simulink model "power_wind_dfig"  (R2016a)
settings: Solver=ode23tb  StartTime=0.0  StopTime=100  FixedStep=1/60  MaxStep=1/60  RelTol=1e-4  AbsTol=1e-3
InitFcn:
  | xInitial = init_power_wind_dfig;
undefined symbols (not defined in the file): b0, D1, D11, Delta, F, find_system, Fnom, gcbh, H, ILd_init, ILq_init, Imax_grid_conv, Init, j, Kd, Ki_dc_reg, Ki_grid_side_cur_reg, Ki_power_reg, Ki_Q, Ki_rotor_side_cur_reg, Ki_volt_reg, Kp, Kp_dc_reg, Kp_grid_side_cur_reg, Kp_power_reg, Kp_Q, Kp_rotor_side_cur_reg, Kp_volt_reg, L_RL, Llr, Lls, p, Pnom, power_A, power_B, power_D, R_RL, Rr, Rs, speed_A, speed_B, speed_C, speed_D, sps_rtmsupport, Vcontrol, Vnom, Wind_On, wo
libraries: powerlib_meascontrol x29, powerlib x27, simulink_extras x5, re_lib x2
(part 4 of 5)

== system power_wind_dfig/Wind Turbine Doubly-Fed Induction Generator (Phasor Type)1/Generator & Converters/Control/wind_dfig_grid/Current regulator ==
  Vdq : Inport
  Idq : Inport  Port=2
  Idq_ref : Inport  Port=3
  Constant1 : Constant  Value=L_RL
  Constant2 : Constant  Value=L_RL
  Constant3 : Constant  Value=R_RL
  Constant4 : Constant  Value=R_RL
  Demux{,1..3} (4 alike) : Demux  Outputs=2
  Mux : Mux  Inputs=2
  Mux1 : Mux  Inputs=2
  Product{,1..3} (4 alike) : Product  SaturateOnIntegerOverflow=on  InputSameDT=on  OutDataTypeStr=Inherit: Same as first input
  Subsystem3 : Subsystem  mask{Kp=Kp_grid_side_cur_reg, Ki=Ki_grid_side_cur_reg, Limits=[inf -inf], Init=0}
      mask prompts: Kp "Proportional gain (Kp):"; Ki "Integral gain (Ki):"; Limits "Output limits [Upper Lower]:"; Init "Output initial value:"
      mask init:
      | Upper_Limit=Limits(1);
      | Lower_Limit=Limits(2);
      mask Display: disp('PI')
  Sum1 : Sum  Inputs=|+-  SaturateOnIntegerOverflow=on  InputSameDT=on  OutDataTypeStr=Inherit: Same as first input
  Sum2 : Sum  Inputs=-+|  SaturateOnIntegerOverflow=on  InputSameDT=on  OutDataTypeStr=Inherit: Same as first input
  Sum3 : Sum  Inputs=||++-  SaturateOnIntegerOverflow=on  InputSameDT=on  OutDataTypeStr=Inherit: Same as first input
  Sum4 : Sum  Inputs=|+-  SaturateOnIntegerOverflow=on  InputSameDT=on  OutDataTypeStr=Inherit: Same as first input
  Sum5 : Sum  Inputs=|--+  SaturateOnIntegerOverflow=on  InputSameDT=on  OutDataTypeStr=Inherit: Same as first input
  Sum6 : Sum  Inputs=|-+  SaturateOnIntegerOverflow=on  InputSameDT=on  OutDataTypeStr=Inherit: Same as first input
  Vdq* : Outport
  wires:
  Constant2/1 -> Product1/2
  Demux3/1 -> Sum1/2  "vd'"
  Subsystem3/1(Out1) -> Demux3/1
  Mux1/1 -> Subsystem3/1(In1)
  Sum5/1 -> Sum6/2
  Sum3/1 -> Sum1/1
  Demux2/1 -> Sum3/1  "Vd"
  Constant1/1 -> Product/1
  Vdq/1 -> Demux2/1
  Demux1/2 -> Sum2/2  "Iq_ref"
  Idq_ref/1 -> Demux1/1
  Demux1/1 -> Sum4/1  "Id_ref"
  Sum2/1 -> Mux1/2
  Demux/2 -> Product/2, Sum2/1, Product3/1  "Iq"
  Demux/1 -> Product1/1, Sum4/2, Product2/2  "Id"
  Idq/1 -> Demux/1
  Sum6/1 -> Mux/2
  Sum1/1 -> Mux/1
  Mux/1 -> Vdq*/1
  Demux3/2 -> Sum6/1  "vq'"
  Product/1 -> Sum3/2
  Sum4/1 -> Mux1/1
  Constant3/1 -> Product2/1
  Constant4/1 -> Product3/2
  Product1/1 -> Sum5/2
  Demux2/2 -> Sum5/3  "Vq"
  Product2/1 -> Sum3/3
  Product3/1 -> Sum5/1

== system power_wind_dfig/Wind Turbine Doubly-Fed Induction Generator (Phasor Type)1/Generator & Converters/Control/wind_dfig_grid/DC bus voltage Regulator ==
  Vdc_ref : Inport
  Vdc : Inport  Port=2
  Rate Limiter : RateLimiter  RisingSlewLimit=current_slew_rate  FallingSlewLimit=-current_slew_rate
  Subsystem1 : Subsystem  mask{Kp=Kp_dc_reg, Ki=Ki_dc_reg, Limits=[1 -1]*Imax_grid_conv, Init=ILd_init}
      mask prompts: Kp "Proportional gain (Kp):"; Ki "Integral gain (Ki):"; Limits "Output limits [Upper Lower]:"; Init "Output initial value:"
      mask init:
      | Upper_Limit=Limits(1);
      | Lower_Limit=Limits(2);
      mask Display: disp('PI')
  Sum7 : Sum  Inputs=|+-  SaturateOnIntegerOverflow=on  InputSameDT=on  OutDataTypeStr=Inherit: Same as first input
  Id_ref : Outport
  wires:
  Rate Limiter/1 -> Id_ref/1
  Vdc/1 -> Sum7/2
  Subsystem1/1(Out1) -> Rate Limiter/1
  Vdc_ref/1 -> Sum7/1
  Sum7/1 -> Subsystem1/1(In1)

== system power_wind_dfig/Wind Turbine Doubly-Fed Induction Generator (Phasor Type)1/Generator & Converters/Control/wind_dfig_grid/Idq B1 voltage Reference frame ==
  Theta : Inport
  Idq_grid_conv : Inport  Port=2
  Complex to Magnitude-Angle : ComplexToMagnitudeAngle
  Complex to Real-Imag : ComplexToRealImag
  Demux1 : Demux  Outputs=2
  Magnitude-Angle to Complex : MagnitudeAngleToComplex
  Mux : Mux  Inputs=2
  Real-Imag to Complex : RealImagToComplex
  Sum : Sum  Inputs=|+-  SaturateOnIntegerOverflow=on
  Idq : Outport
  wires:
  Complex to Real-Imag/2 -> Mux/2  "Iq"
  Complex to Real-Imag/1 -> Mux/1  "Id"
  Magnitude-Angle to Complex/1 -> Complex to Real-Imag/1
  Sum/1 -> Magnitude-Angle to Complex/2
  Complex to Magnitude-Angle/1 -> Magnitude-Angle to Complex/1
  Complex to Magnitude-Angle/2 -> Sum/1
  Mux/1 -> Idq/1
  Idq_grid_conv/1 -> Demux1/1
  Demux1/1 -> Real-Imag to Complex/1
  Demux1/2 -> Real-Imag to Complex/2
  Real-Imag to Complex/1 -> Complex to Magnitude-Angle/1
  Theta/1 -> Sum/2

== system power_wind_dfig/Wind Turbine Doubly-Fed Induction Generator (Phasor Type)1/Generator & Converters/Control/wind_dfig_grid/Idq references ==
  Id*Iq* : Inport
  Cartesian to Polar : simulink_extras/Transformations/Cartesian to Polar
  Demux : Demux  Outputs=2
  Igrid_conv_max^2 : Constant  Value=Imax_grid_conv*Imax_grid_conv
  Math Function : Math  Operator=square  SaturateOnIntegerOverflow=on
  Math Function1 : Math  Operator=sqrt  SaturateOnIntegerOverflow=on
  Mux : Mux  Inputs=2
  Mux1 : Mux  Inputs=2
  Product : Product  SaturateOnIntegerOverflow=on  InputSameDT=on  OutDataTypeStr=Inherit: Same as first input
  Rate Limiter : RateLimiter  RisingSlewLimit=current_slew_rate  FallingSlewLimit=-current_slew_rate
  Sign : Signum  ZeroCross=off
  Sum : Sum  Inputs=|+-  SaturateOnIntegerOverflow=on  InputSameDT=on  OutDataTypeStr=Inherit: Same as first input
  Switch : Switch  Threshold=Imax_grid_conv  SaturateOnIntegerOverflow=on  InputSameDT=on
  Terminator : Terminator
  Idq_ref : Outport
  wires:
  Id*Iq*/1 -> Demux/1
  Sign/1 -> Product/1
  Math Function1/1 -> Product/2  "Iq"
  Switch/1 -> Rate Limiter/1
  Mux1/1 -> Switch/1
  Sum/1 -> Math Function1/1
  Math Function/1 -> Sum/2
  Igrid_conv_max^2/1 -> Sum/1
  Mux/1 -> Switch/3
  Cartesian to Polar/1 -> Switch/2
  Cartesian to Polar/2 -> Terminator/1
  Demux/1 -> Mux/1, Cartesian to Polar/1, Math Function/1, Mux1/1
  Demux/2 -> Sign/1, Mux/2, Cartesian to Polar/2
  Rate Limiter/1 -> Idq_ref/1
  Product/1 -> Mux1/2

== system power_wind_dfig/Wind Turbine Doubly-Fed Induction Generator (Phasor Type)1/Generator & Converters/Control/wind_dfig_grid/Subsystem ==
  note: Where Vnom = RMS ph-ph nominal voltage
  note: m = Vnom * 2*sqrt(2/3) / Vdc
  note: Required value for modulation index "m" to obtain 1 pu generated voltage by the converter:
  Theta : Inport
  Vdq* : Inport  Port=2
  Vdc : Inport  Port=3
  0-1 : Saturate  UpperLimit=1  LowerLimit=0
  Avoid division by zero : Saturate  UpperLimit=1e6  LowerLimit=1e-6
  Cartesian to Polar1 : simulink_extras/Transformations/Cartesian to Polar
  Demux1 : Demux  Outputs=2
  K : Constant  Value=Vnom*2*sqrt(2/3)
  Magnitude-Angle to Complex : MagnitudeAngleToComplex
  Product1 : Product  Inputs=**/  SaturateOnIntegerOverflow=on  InputSameDT=on  OutDataTypeStr=Inherit: Same as first input
  Sum : Sum  Inputs=|++  SaturateOnIntegerOverflow=on
  Vdq_ctrl_grid_conv : Outport
  wires:
  Cartesian to Polar1/2 -> Sum/1
  Cartesian to Polar1/1 -> Product1/1
  Demux1/2 -> Cartesian to Polar1/2
  Demux1/1 -> Cartesian to Polar1/1
  Vdq*/1 -> Demux1/1
  Avoid division by zero/1 -> Product1/3
  K/1 -> Product1/2
  Vdc/1 -> Avoid division by zero/1
  Product1/1 -> 0-1/1  "m"
  0-1/1 -> Magnitude-Angle to Complex/1
  Sum/1 -> Magnitude-Angle to Complex/2
  Magnitude-Angle to Complex/1 -> Vdq_ctrl_grid_conv/1
  Theta/1 -> Sum/2

== system power_wind_dfig/Wind Turbine Doubly-Fed Induction Generator (Phasor Type)1/Generator & Converters/Control/wind_dfig_grid/Vdq B1 voltage Reference frame ==
  Theta : Inport
  Vdq_B1 : Inport  Port=2
  Complex to Magnitude-Angle : ComplexToMagnitudeAngle
  Complex to Real-Imag : ComplexToRealImag
  Demux1 : Demux  Outputs=2
  Magnitude-Angle to Complex : MagnitudeAngleToComplex
  Mux : Mux  Inputs=2
  Real-Imag to Complex : RealImagToComplex
  Sum : Sum  Inputs=|+-  SaturateOnIntegerOverflow=on
  Vdq : Outport
  wires:
  Complex to Real-Imag/2 -> Mux/2  "Vq"
  Complex to Real-Imag/1 -> Mux/1  "Vd"
  Magnitude-Angle to Complex/1 -> Complex to Real-Imag/1
  Sum/1 -> Magnitude-Angle to Complex/2
  Complex to Magnitude-Angle/1 -> Magnitude-Angle to Complex/1
  Complex to Magnitude-Angle/2 -> Sum/1
  Mux/1 -> Vdq/1
  Vdq_B1/1 -> Demux1/1
  Demux1/1 -> Real-Imag to Complex/1
  Demux1/2 -> Real-Imag to Complex/2
  Real-Imag to Complex/1 -> Complex to Magnitude-Angle/1
  Theta/1 -> Sum/2

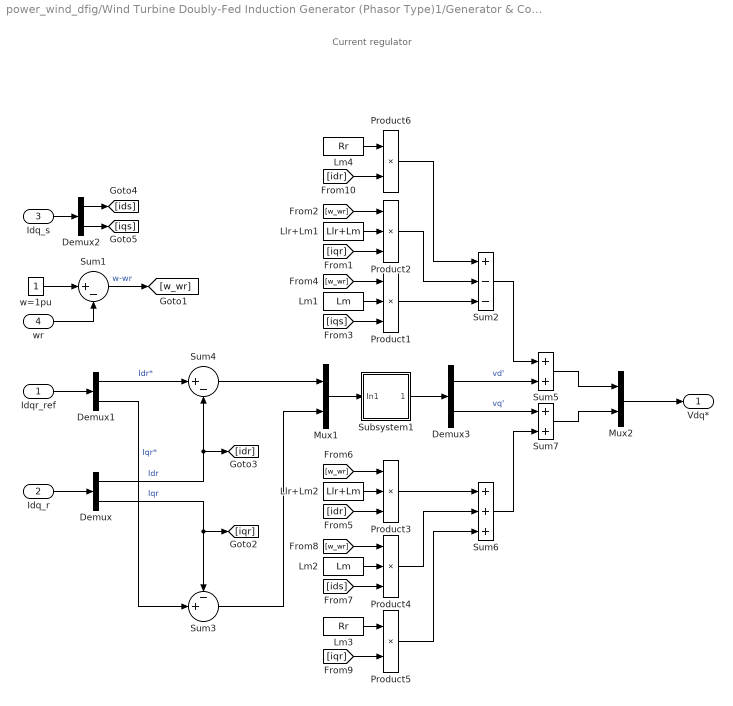
== system power_wind_dfig/Wind Turbine Doubly-Fed Induction Generator (Phasor Type)1/Generator & Converters/Control/wind_dfig_rotor/Current Regulator ==
  note: Current regulator
  Idqr_ref : Inport
  Idq_r : Inport  Port=2
  Idq_s : Inport  Port=3
  wr : Inport  Port=4
  Demux{,1..3} (4 alike) : Demux  Outputs=2
  Llr+Lm1 : Constant  Value=Llr+Lm
  Llr+Lm2 : Constant  Value=Llr+Lm
  Lm1 : Constant  Value=Lm
  Lm2 : Constant  Value=Lm
  Lm3 : Constant  Value=Rr
  Lm4 : Constant  Value=Rr
  Mux1 : Mux  Inputs=2
  Mux2 : Mux  Inputs=2
  Product{1..4} (4 alike) : Product  Inputs=3  SaturateOnIntegerOverflow=on  OutDataTypeStr=Inherit: Same as first input
  Product5 : Product  SaturateOnIntegerOverflow=on  OutDataTypeStr=Inherit: Same as first input
  Product6 : Product  SaturateOnIntegerOverflow=on  OutDataTypeStr=Inherit: Same as first input
  Subsystem1 : Subsystem  mask{Kp=Kp_rotor_side_cur_reg, Ki=Ki_rotor_side_cur_reg, Limits=[inf -inf], Init=0}
      mask prompts: Kp "Proportional gain (Kp):"; Ki "Integral gain (Ki):"; Limits "Output limits [Upper Lower]:"; Init "Output initial value:"
      mask init:
      | Upper_Limit=Limits(1);
      | Lower_Limit=Limits(2);
      mask Display: disp('PI')
  Sum1 : Sum  Inputs=|+-  SaturateOnIntegerOverflow=on  InputSameDT=on  OutDataTypeStr=Inherit: Same as first input
  Sum2 : Sum  Inputs=+--  SaturateOnIntegerOverflow=on  InputSameDT=on  OutDataTypeStr=Inherit: Same as first input
  Sum3 : Sum  Inputs=-+|  SaturateOnIntegerOverflow=on  InputSameDT=on  OutDataTypeStr=Inherit: Same as first input
  Sum4 : Sum  Inputs=|+-  SaturateOnIntegerOverflow=on  InputSameDT=on  OutDataTypeStr=Inherit: Same as first input
  Sum5 : Sum  SaturateOnIntegerOverflow=on  InputSameDT=on  OutDataTypeStr=Inherit: Same as first input
  Sum6 : Sum  Inputs=+++  SaturateOnIntegerOverflow=on  InputSameDT=on  OutDataTypeStr=Inherit: Same as first input
  Sum7 : Sum  SaturateOnIntegerOverflow=on  InputSameDT=on  OutDataTypeStr=Inherit: Same as first input
  w=1pu : Constant
  Vdq* : Outport
  wires:
  Product5/1 -> Sum6/3
  Product6/1 -> Sum2/1
  Product1/1 -> Sum2/3
  Product2/1 -> Sum2/2
  [idr] -> Product6/2
  Lm4/1 -> Product6/1
  [iqr] -> Product5/2
  Lm3/1 -> Product5/1
  Sum2/1 -> Sum5/1
  Sum6/1 -> Sum7/2
  Product4/1 -> Sum6/2
  Mux2/1 -> Vdq*/1
  Sum7/1 -> Mux2/2
  Sum5/1 -> Mux2/1
  Demux3/2 -> Sum7/1  "vq'"
  Product3/1 -> Sum6/1
  Lm2/1 -> Product4/2
  [w_wr] -> Product4/1
  [ids] -> Product4/3
  Llr+Lm2/1 -> Product3/2
  [w_wr] -> Product3/1
  [idr] -> Product3/3
  Lm1/1 -> Product1/2
  [w_wr] -> Product1/1
  [iqs] -> Product1/3
  Llr+Lm1/1 -> Product2/2
  [w_wr] -> Product2/1
  [iqr] -> Product2/3
  Sum1/1 -> [w_wr]  "w-wr"
  Demux2/2 -> [iqs]
  Demux2/1 -> [ids]
  Demux3/1 -> Sum5/2  "vd'"
  wr/1 -> Sum1/2
  w=1pu/1 -> Sum1/1
  Subsystem1/1(Out1) -> Demux3/1
  Idq_s/1 -> Demux2/1
  Mux1/1 -> Subsystem1/1(In1)
  Demux1/2 -> Sum3/2  "Iqr*"
  Demux1/1 -> Sum4/1  "Idr*"
  Idqr_ref/1 -> Demux1/1
  Sum3/1 -> Mux1/2
  Sum4/1 -> Mux1/1
  Demux/2 -> [iqr], Sum3/1  "Iqr"
  Demux/1 -> [idr], Sum4/2  "Idr"
  Idq_r/1 -> Demux/1

== system power_wind_dfig/Wind Turbine Doubly-Fed Induction Generator (Phasor Type)1/Generator & Converters/Control/wind_dfig_rotor/Idq B1 voltage Reference frame ==
  Theta : Inport
  Idq_rotor : Inport  Port=2
  Idq_stator : Inport  Port=3
  Idq_grid_conv : Inport  Port=4
  Complex to Magnitude-Angle : ComplexToMagnitudeAngle
  Complex to Magnitude-Angle1 : ComplexToMagnitudeAngle
  Complex to Magnitude-Angle2 : ComplexToMagnitudeAngle
  Complex to Real-Imag : ComplexToRealImag
  Complex to Real-Imag1 : ComplexToRealImag
  Complex to Real-Imag2 : ComplexToRealImag
  Demux : Demux  Outputs=2
  Demux1 : Demux  Outputs=2
  Demux2 : Demux  Outputs=2
  Magnitude-Angle to Complex : MagnitudeAngleToComplex
  Magnitude-Angle to Complex1 : MagnitudeAngleToComplex
  Magnitude-Angle to Complex2 : MagnitudeAngleToComplex
  Mux : Mux  Inputs=2
  Mux1 : Mux  Inputs=2
  Mux2 : Mux  Inputs=2
  Real-Imag to Complex : RealImagToComplex
  Real-Imag to Complex1 : RealImagToComplex
  Real-Imag to Complex2 : RealImagToComplex
  Sum : Sum  Inputs=|+-  SaturateOnIntegerOverflow=on
  Sum1 : Sum  Inputs=|+-  SaturateOnIntegerOverflow=on
  Sum2 : Sum  Inputs=|+-  SaturateOnIntegerOverflow=on
  Idq_r : Outport
  Idq_s : Outport  Port=2
  Idq_gc : Outport  Port=3
  wires:
  Idq_grid_conv/1 -> Demux2/1
  Demux2/2 -> Real-Imag to Complex2/2
  Demux2/1 -> Real-Imag to Complex2/1
  Mux2/1 -> Idq_gc/1
  Real-Imag to Complex2/1 -> Complex to Magnitude-Angle2/1
  Complex to Magnitude-Angle2/2 -> Sum2/1
  Complex to Magnitude-Angle2/1 -> Magnitude-Angle to Complex2/1
  Sum2/1 -> Magnitude-Angle to Complex2/2
  Magnitude-Angle to Complex2/1 -> Complex to Real-Imag2/1
  Complex to Real-Imag2/1 -> Mux2/1
  Complex to Real-Imag2/2 -> Mux2/2
  Theta/1 -> Sum2/2, Sum1/2, Sum/2
  Idq_rotor/1 -> Demux1/1
  Demux1/2 -> Real-Imag to Complex1/2
  Demux1/1 -> Real-Imag to Complex1/1
  Mux1/1 -> Idq_r/1
  Real-Imag to Complex1/1 -> Complex to Magnitude-Angle1/1
  Complex to Magnitude-Angle1/2 -> Sum1/1
  Complex to Magnitude-Angle1/1 -> Magnitude-Angle to Complex1/1
  Sum1/1 -> Magnitude-Angle to Complex1/2
  Magnitude-Angle to Complex1/1 -> Complex to Real-Imag1/1
  Complex to Real-Imag1/1 -> Mux1/1
  Complex to Real-Imag1/2 -> Mux1/2
  Idq_stator/1 -> Demux/1
  Demux/2 -> Real-Imag to Complex/2
  Demux/1 -> Real-Imag to Complex/1
  Mux/1 -> Idq_s/1
  Real-Imag to Complex/1 -> Complex to Magnitude-Angle/1
  Complex to Magnitude-Angle/2 -> Sum/1
  Complex to Magnitude-Angle/1 -> Magnitude-Angle to Complex/1
  Sum/1 -> Magnitude-Angle to Complex/2
  Magnitude-Angle to Complex/1 -> Complex to Real-Imag/1
  Complex to Real-Imag/1 -> Mux/1
  Complex to Real-Imag/2 -> Mux/2

== system power_wind_dfig/Wind Turbine Doubly-Fed Induction Generator (Phasor Type)1/Generator & Converters/Control/wind_dfig_rotor/Idq Mutual flux Reference frame ==
  angle_flux : Inport
  Idq_r : Inport  Port=2
  Idq_s : Inport  Port=3
  Complex to Magnitude-Angle : ComplexToMagnitudeAngle
  Complex to Magnitude-Angle1 : ComplexToMagnitudeAngle
  Complex to Real-Imag : ComplexToRealImag
  Complex to Real-Imag1 : ComplexToRealImag
  Demux : Demux  Outputs=2
  Demux1 : Demux  Outputs=2
  Magnitude-Angle to Complex : MagnitudeAngleToComplex
  Magnitude-Angle to Complex1 : MagnitudeAngleToComplex
  Mux : Mux  Inputs=2
  Mux1 : Mux  Inputs=2
  Real-Imag to Complex : RealImagToComplex
  Real-Imag to Complex1 : RealImagToComplex
  Sum : Sum  Inputs=|+-  SaturateOnIntegerOverflow=on
  Sum1 : Sum  Inputs=|+-  SaturateOnIntegerOverflow=on
  "Idq_r " : Outport
  "Idq_s " : Outport  Port=2
  wires:
  Real-Imag to Complex1/1 -> Complex to Magnitude-Angle1/1
  Demux1/2 -> Real-Imag to Complex1/2
  Demux1/1 -> Real-Imag to Complex1/1
  Idq_s/1 -> Demux1/1
  Magnitude-Angle to Complex1/1 -> Complex to Real-Imag1/1
  Sum1/1 -> Magnitude-Angle to Complex1/2
  Complex to Magnitude-Angle1/1 -> Magnitude-Angle to Complex1/1
  Complex to Magnitude-Angle1/2 -> Sum1/1
  Mux1/1 -> "Idq_s "/1
  Complex to Real-Imag1/1 -> Mux1/1
  Complex to Real-Imag1/2 -> Mux1/2
  Real-Imag to Complex/1 -> Complex to Magnitude-Angle/1
  Demux/2 -> Real-Imag to Complex/2
  Demux/1 -> Real-Imag to Complex/1
  Idq_r/1 -> Demux/1
  Magnitude-Angle to Complex/1 -> Complex to Real-Imag/1
  Sum/1 -> Magnitude-Angle to Complex/2
  Complex to Magnitude-Angle/1 -> Magnitude-Angle to Complex/1
  angle_flux/1 -> Sum1/2, Sum/2
  Complex to Magnitude-Angle/2 -> Sum/1
  Mux/1 -> "Idq_r "/1
  Complex to Real-Imag/1 -> Mux/1
  Complex to Real-Imag/2 -> Mux/2

== system power_wind_dfig/Wind Turbine Doubly-Fed Induction Generator (Phasor Type)1/Generator & Converters/Control/wind_dfig_rotor/Mutual flux ==
  Idq_r : Inport
  Idq_s : Inport  Port=2
  20% : Switch  Threshold=0.5  SaturateOnIntegerOverflow=on
  Cartesian to Polar : simulink_extras/Transformations/Cartesian to Polar
  Constant1 : Constant  Value=Lm
  Demux : Demux  Outputs=2
  Demux1 : Demux  Outputs=2
  IC=ic : Memory  X0=-pi/2  InheritSampleTime=on
  Product1 : Product  SaturateOnIntegerOverflow=on  InputSameDT=on  OutDataTypeStr=Inherit: Same as first input
  Product5 : Product  SaturateOnIntegerOverflow=on  InputSameDT=on  OutDataTypeStr=Inherit: Same as first input
  Relay : Relay  OnSwitchValue=0.5  OffSwitchValue=0.1
  Sum1 : Sum  SaturateOnIntegerOverflow=on  InputSameDT=on  OutDataTypeStr=Inherit: Same as first input
  Sum2 : Sum  SaturateOnIntegerOverflow=on  InputSameDT=on  OutDataTypeStr=Inherit: Same as first input
  angle_fluxm : Outport
  wires:
  Cartesian to Polar/2 -> 20%/1  "angle_phi"
  Relay/1 -> 20%/2
  20%/1 -> angle_fluxm/1, IC=ic/1
  IC=ic/1 -> 20%/3
  Idq_r/1 -> Demux/1
  Idq_s/1 -> Demux1/1
  Product1/1 -> Cartesian to Polar/1  "phidm"
  Constant1/1 -> Product5/1, Product1/1
  Sum2/1 -> Product5/2  "iqm"
  Demux/2 -> Sum2/2
  Demux1/2 -> Sum2/1
  Sum1/1 -> Product1/2  "idm"
  Demux/1 -> Sum1/2
  Demux1/1 -> Sum1/1
  Product5/1 -> Cartesian to Polar/2  "phiqm"
  Cartesian to Polar/1 -> Relay/1  "mod_phi"

== system power_wind_dfig/Wind Turbine Doubly-Fed Induction Generator (Phasor Type)1/Generator & Converters/Control/wind_dfig_rotor/Power Regulator ==
  Pelec : Inport
  wr : Inport  Port=2
  idqr : Inport  Port=3
  idqs : Inport  Port=4
  idq_grid_conv : Inport  Port=5
  Power_opt : Inport  Port=6
  ExternalTorque : Constant  Value=Wind_On
  Logical Operator : Logic  Operator=NOT  AllPortsSameDT=off
  Rate Limiter : RateLimiter  RisingSlewLimit=current_slew_rate  FallingSlewLimit=-current_slew_rate
  Saturation : Saturate  UpperLimit=1  LowerLimit=0
  Subsystem : Subsystem
  "Subsystem " : Subsystem
  Switch : Switch  Threshold=0.5  SaturateOnIntegerOverflow=on
  Iqr* : Outport
  wires:
  Power_opt/1 -> "Subsystem "/3(Power_opt)
  idq_grid_conv/1 -> Subsystem/5(idq_grid_conv)
  idqr/1 -> "Subsystem "/2(idqr), Subsystem/4(idqr)
  idqs/1 -> Subsystem/3(idqs)
  Rate Limiter/1 -> Iqr*/1
  "Subsystem "/1(Iqr*) -> Switch/3
  Subsystem/1(Iqr*) -> Switch/1
  ExternalTorque/1 -> Logical Operator/1, Subsystem/Enable, Switch/2
  Switch/1 -> Saturation/1
  Saturation/1 -> Rate Limiter/1
  Pelec/1 -> "Subsystem "/1(Pelec), Subsystem/1(Pelec)
  wr/1 -> Subsystem/2(wr)
  Logical Operator/1 -> "Subsystem "/Enable

== system power_wind_dfig/Wind Turbine Doubly-Fed Induction Generator (Phasor Type)1/Generator & Converters/Control/wind_dfig_rotor/Priority Idr ==
  Idqr* : Inport
  Cartesian to Polar : simulink_extras/Transformations/Cartesian to Polar
  Demux : Demux  Outputs=2
  Irotor_max^2 : Constant
  Math Function : Math  Operator=square  SaturateOnIntegerOverflow=on
  Math Function1 : Math  Operator=sqrt  SaturateOnIntegerOverflow=on
  Mux : Mux  Inputs=2
  Mux1 : Mux  Inputs=2
  Product : Product  SaturateOnIntegerOverflow=on  InputSameDT=on  OutDataTypeStr=Inherit: Same as first input
  Rate Limiter : RateLimiter  RisingSlewLimit=current_slew_rate  FallingSlewLimit=-current_slew_rate
  Sign : Signum  ZeroCross=off
  Sum : Sum  Inputs=|+-  SaturateOnIntegerOverflow=on  InputSameDT=on  OutDataTypeStr=Inherit: Same as first input
  Switch : Switch  Threshold=1  SaturateOnIntegerOverflow=on  InputSameDT=on
  Terminator : Terminator
  Idqr_ref : Outport
  wires:
  Idqr*/1 -> Demux/1
  Rate Limiter/1 -> Idqr_ref/1
  Sign/1 -> Product/1
  Math Function1/1 -> Product/2
  Switch/1 -> Rate Limiter/1
  Mux1/1 -> Switch/1
  Sum/1 -> Math Function1/1
  Math Function/1 -> Sum/2
  Irotor_max^2/1 -> Sum/1
  Mux/1 -> Switch/3
  Cartesian to Polar/1 -> Switch/2
  Cartesian to Polar/2 -> Terminator/1
  Demux/1 -> Mux/1, Cartesian to Polar/1, Math Function/1, Mux1/1
  Demux/2 -> Sign/1, Mux/2, Cartesian to Polar/2
  Product/1 -> Mux1/2

== system power_wind_dfig/Wind Turbine Doubly-Fed Induction Generator (Phasor Type)1/Generator & Converters/Control/wind_dfig_rotor/Q Regulator ==
  Q_ref : Inport
  Q_B1 : Inport  Port=2
  Idr_init : Inport  Port=3
  Enable : EnablePort  PropagateVarSize=During execution  ZeroCross=off
  Mean Value : Subsystem  mask(Mean value){Period=1/Fnom}
      mask prompts: Period "Averaging period (s):"
      mask help: This block uses the running window averaging technique to compute the mean value of the input signal over the specified period.
  Rate Limiter : RateLimiter  RisingSlewLimit=current_slew_rate  FallingSlewLimit=-current_slew_rate
  "Rate Limiter " : RateLimiter  RisingSlewLimit=Q_slew_rate  FallingSlewLimit=-Q_slew_rate
  Subsystem1 : Subsystem  mask{Kp=Kp_Q, Ki=Ki_Q, Limits=[1 -1]}
      mask prompts: Kp "Proportional gain (Kp):"; Ki "Integral gain (Ki):"; Limits "Output limits [Upper Lower]:"
      mask init:
      | Upper_Limit=Limits(1);
      | Lower_Limit=Limits(2);
      mask Display: disp('PI')
  Sum : Sum  Inputs=|+-  SaturateOnIntegerOverflow=on  InputSameDT=on  OutDataTypeStr=Inherit: Same as first input
  Idr* : Outport
  wires:
  Idr_init/1 -> Subsystem1/2(Init)
  Mean Value/1(Mean) -> Sum/2
  Q_B1/1 -> Mean Value/1(In)
  "Rate Limiter "/1 -> Sum/1, Mean Value/2(Init)
  Rate Limiter/1 -> Idr*/1
  Q_ref/1 -> "Rate Limiter "/1
  Sum/1 -> Subsystem1/1(In1)
  Subsystem1/1(Out1) -> Rate Limiter/1  "Idr*"

== system power_wind_dfig/Wind Turbine Doubly-Fed Induction Generator (Phasor Type)1/Generator & Converters/Control/wind_dfig_rotor/V Regulator ==
  V_ref : Inport
  V_B1 : Inport  Port=2
  Idr_init : Inport  Port=3
  Idq_stator : Inport  Port=4
  Idq_grid_conv : Inport  Port=5
  Enable : EnablePort  PropagateVarSize=During execution  ZeroCross=off
  Droop : Gain  Gain=Xs  SaturateOnIntegerOverflow=on  OutDataTypeStr=Inherit: Same as input  ParamDataTypeStr=Inherit: Same as input
  Mean Value : Subsystem  mask(Mean value){Period=1/Fnom}
      mask prompts: Period "Averaging period (s):"
      mask help: This block uses the running window averaging technique to compute the mean value of the input signal over the specified period.
  Mean Value1 : Subsystem  mask(Mean value){Period=1/Fnom}
      mask prompts: Period "Averaging period (s):"
      mask help: This block uses the running window averaging technique to compute the mean value of the input signal over the specified period.
  Rate Limiter : RateLimiter  RisingSlewLimit=current_slew_rate  FallingSlewLimit=-current_slew_rate
  "Rate Limiter " : RateLimiter  RisingSlewLimit=V_slew_rate  FallingSlewLimit=-V_slew_rate
  Selector1 : Selector  InputPortWidth=2  IndexOptions=Index vector (dialog)  Indices=2  OutputSizes=1
  Selector2 : Selector  InputPortWidth=2  IndexOptions=Index vector (dialog)  Indices=2  OutputSizes=1
  Subsystem1 : Subsystem  mask{Kp=Kp_volt_reg, Ki=Ki_volt_reg, Limits=[1 -1]}
      mask prompts: Kp "Proportional gain (Kp):"; Ki "Integral gain (Ki):"; Limits "Output limits [Upper Lower]:"
      mask init:
      | Upper_Limit=Limits(1);
      | Lower_Limit=Limits(2);
      mask Display: disp('PI')
  Sum : Sum  Inputs=|-+-  SaturateOnIntegerOverflow=on  InputSameDT=on  OutDataTypeStr=Inherit: Same as first input
  Sum1 : Sum  SaturateOnIntegerOverflow=on  InputSameDT=on  OutDataTypeStr=Inherit: Same as first input
  Idr* : Outport
  wires:
  Mean Value1/1(Mean) -> Sum/1
  Idr_init/1 -> Subsystem1/2(Init)
  Droop/1 -> Mean Value1/2(Init), Mean Value1/1(In)
  Sum1/1 -> Droop/1
  Selector2/1 -> Sum1/2
  Selector1/1 -> Sum1/1
  Idq_grid_conv/1 -> Selector2/1
  Idq_stator/1 -> Selector1/1
  V_B1/1 -> Mean Value/1(In)
  Mean Value/1(Mean) -> Sum/3
  Subsystem1/1(Out1) -> Rate Limiter/1  "Idr*"
  Sum/1 -> Subsystem1/1(In1)
  V_ref/1 -> "Rate Limiter "/1
  Rate Limiter/1 -> Idr*/1
  "Rate Limiter "/1 -> Sum/2, Mean Value/2(Init)

== system power_wind_dfig/Wind Turbine Doubly-Fed Induction Generator (Phasor Type)1/Generator & Converters/Control/wind_dfig_rotor/dq --> abc ==
  note: Required value for modulation index "m" to obtain 1 pu generated voltage by the converter:
  note: m = Vnom * 2*sqrt(2/3) / Vdc
  note: Where Vnom = RMS ph-ph nominal voltage
  Vdq* : Inport
  Vdc : Inport  Port=2
  Angle : Inport  Port=3
  0-1 : Saturate  UpperLimit=1  LowerLimit=0
  Avoid division by zero : Saturate  UpperLimit=1e6  LowerLimit=1e-6
  Cartesian to Polar : simulink_extras/Transformations/Cartesian to Polar
  Demux1 : Demux  Outputs=2
  K : Constant  Value=Vnom*2*sqrt(2/3)
  Magnitude-Angle to Complex : MagnitudeAngleToComplex
  Product2 : Product  Inputs=**/  SaturateOnIntegerOverflow=on  InputSameDT=on  OutDataTypeStr=Inherit: Same as first input
  Sum : Sum  Inputs=|++  SaturateOnIntegerOverflow=on
  Vdq_ctrl_rotor_conv : Outport
  wires:
  Magnitude-Angle to Complex/1 -> Vdq_ctrl_rotor_conv/1
  Angle/1 -> Sum/2
  Sum/1 -> Magnitude-Angle to Complex/2
  0-1/1 -> Magnitude-Angle to Complex/1
  Product2/1 -> 0-1/1  "m"
  Vdc/1 -> Avoid division by zero/1
  K/1 -> Product2/2
  Avoid division by zero/1 -> Product2/3
  Demux1/1 -> Cartesian to Polar/1
  Demux1/2 -> Cartesian to Polar/2
  Cartesian to Polar/1 -> Product2/1
  Cartesian to Polar/2 -> Sum/1
  Vdq*/1 -> Demux1/1

== system power_wind_dfig/Wind Turbine Protection/Protection System/AC Current Protection/Current Measurement/magnitude ==
  In1 : Inport
  Complex to Real-Imag : ComplexToRealImag
  Fourier1 : Subsystem  mask(Fourier analyser){f1=Freq, n=0}
      mask prompts: f1 "Fundamental frequency f1 (Hz):"; n "Harmonic n (0=DC; 1=fundamental; 2=2nd harm;  ...) :"
      mask help: The Fourier block performs a Fourier analysis of the input signal over a running window of one cycle of the fundamental frequency. First and second outputs return respectively the magnitude and phase (degrees) of the harmonic component specified.
      mask init:
      | k=2-(n==0);
      mask Help: helpview(psbhelp)
  Fourier2 : Subsystem  mask(Fourier analyser){f1=Freq, n=0}
      mask prompts: f1 "Fundamental frequency f1 (Hz):"; n "Harmonic n (0=DC; 1=fundamental; 2=2nd harm;  ...) :"
      mask help: The Fourier block performs a Fourier analysis of the input signal over a running window of one cycle of the fundamental frequency. First and second outputs return respectively the magnitude and phase (degrees) of the harmonic component specified.
      mask init:
      | k=2-(n==0);
      mask Help: helpview(psbhelp)
  Math Function : Math  Operator=hypot  SaturateOnIntegerOverflow=on
  Terminator : Terminator
  Terminator1 : Terminator
  Out1 : Outport
  wires:
  Complex to Real-Imag/1 -> Fourier1/1(signal)
  Complex to Real-Imag/2 -> Fourier2/1(signal)
  Fourier1/2(angle) -> Terminator/1
  Fourier2/2(angle) -> Terminator1/1
  Fourier1/1(magnitude) -> Math Function/1
  Fourier2/1(magnitude) -> Math Function/2
  Math Function/1 -> Out1/1
  In1/1 -> Complex to Real-Imag/1

== system power_wind_dfig/Wind Turbine Protection/Protection System/AC Current Protection/Current Measurement/magnitude1 ==
  In1 : Inport
  Complex to Real-Imag : ComplexToRealImag
  Fourier1 : Subsystem  mask(Fourier analyser){f1=Freq, n=0}
      mask prompts: f1 "Fundamental frequency f1 (Hz):"; n "Harmonic n (0=DC; 1=fundamental; 2=2nd harm;  ...) :"
      mask help: The Fourier block performs a Fourier analysis of the input signal over a running window of one cycle of the fundamental frequency. First and second outputs return respectively the magnitude and phase (degrees) of the harmonic component specified.
      mask init:
      | k=2-(n==0);
      mask Help: helpview(psbhelp)
  Fourier2 : Subsystem  mask(Fourier analyser){f1=Freq, n=0}
      mask prompts: f1 "Fundamental frequency f1 (Hz):"; n "Harmonic n (0=DC; 1=fundamental; 2=2nd harm;  ...) :"
      mask help: The Fourier block performs a Fourier analysis of the input signal over a running window of one cycle of the fundamental frequency. First and second outputs return respectively the magnitude and phase (degrees) of the harmonic component specified.
      mask init:
      | k=2-(n==0);
      mask Help: helpview(psbhelp)
  Math Function : Math  Operator=hypot  SaturateOnIntegerOverflow=on
  Terminator : Terminator
  Terminator1 : Terminator
  Out1 : Outport
  wires:
  In1/1 -> Complex to Real-Imag/1
  Math Function/1 -> Out1/1
  Fourier2/1(magnitude) -> Math Function/2
  Fourier1/1(magnitude) -> Math Function/1
  Fourier2/2(angle) -> Terminator1/1
  Fourier1/2(angle) -> Terminator/1
  Complex to Real-Imag/2 -> Fourier2/1(signal)
  Complex to Real-Imag/1 -> Fourier1/1(signal)

== system power_wind_dfig/Wind Turbine Protection/Protection System/AC Voltage Protection/Voltage Measurement/magnitude ==
  In1 : Inport
  Complex to Real-Imag : ComplexToRealImag
  Fourier1 : Subsystem  mask(Fourier analyser){f1=Freq, n=0}
      mask prompts: f1 "Fundamental frequency f1 (Hz):"; n "Harmonic n (0=DC; 1=fundamental; 2=2nd harm;  ...) :"
      mask help: The Fourier block performs a Fourier analysis of the input signal over a running window of one cycle of the fundamental frequency. First and second outputs return respectively the magnitude and phase (degrees) of the harmonic component specified.
      mask init:
      | k=2-(n==0);
      mask Help: helpview(psbhelp)
  Fourier2 : Subsystem  mask(Fourier analyser){f1=Freq, n=0}
      mask prompts: f1 "Fundamental frequency f1 (Hz):"; n "Harmonic n (0=DC; 1=fundamental; 2=2nd harm;  ...) :"
      mask help: The Fourier block performs a Fourier analysis of the input signal over a running window of one cycle of the fundamental frequency. First and second outputs return respectively the magnitude and phase (degrees) of the harmonic component specified.
      mask init:
      | k=2-(n==0);
      mask Help: helpview(psbhelp)
  Math Function : Math  Operator=hypot  SaturateOnIntegerOverflow=on
  Terminator : Terminator
  Terminator1 : Terminator
  Out1 : Outport
  wires:
  Complex to Real-Imag/1 -> Fourier1/1(signal)
  Complex to Real-Imag/2 -> Fourier2/1(signal)
  Fourier1/2(angle) -> Terminator/1
  Fourier2/2(angle) -> Terminator1/1
  Fourier1/1(magnitude) -> Math Function/1
  Fourier2/1(magnitude) -> Math Function/2
  Math Function/1 -> Out1/1
  In1/1 -> Complex to Real-Imag/1

== system power_wind_dfig/Wind Turbine Protection/Protection System/AC Voltage Protection/Voltage Measurement/magnitude1 ==
  In1 : Inport
  Complex to Real-Imag : ComplexToRealImag
  Fourier1 : Subsystem  mask(Fourier analyser){f1=Freq, n=0}
      mask prompts: f1 "Fundamental frequency f1 (Hz):"; n "Harmonic n (0=DC; 1=fundamental; 2=2nd harm;  ...) :"
      mask help: The Fourier block performs a Fourier analysis of the input signal over a running window of one cycle of the fundamental frequency. First and second outputs return respectively the magnitude and phase (degrees) of the harmonic component specified.
      mask init:
      | k=2-(n==0);
      mask Help: helpview(psbhelp)
  Fourier2 : Subsystem  mask(Fourier analyser){f1=Freq, n=0}
      mask prompts: f1 "Fundamental frequency f1 (Hz):"; n "Harmonic n (0=DC; 1=fundamental; 2=2nd harm;  ...) :"
      mask help: The Fourier block performs a Fourier analysis of the input signal over a running window of one cycle of the fundamental frequency. First and second outputs return respectively the magnitude and phase (degrees) of the harmonic component specified.
      mask init:
      | k=2-(n==0);
      mask Help: helpview(psbhelp)
  Math Function : Math  Operator=hypot  SaturateOnIntegerOverflow=on
  Terminator : Terminator
  Terminator1 : Terminator
  Out1 : Outport
  wires:
  In1/1 -> Complex to Real-Imag/1
  Math Function/1 -> Out1/1
  Fourier2/1(magnitude) -> Math Function/2
  Fourier1/1(magnitude) -> Math Function/1
  Fourier2/2(angle) -> Terminator1/1
  Fourier1/2(angle) -> Terminator/1
  Complex to Real-Imag/2 -> Fourier2/1(signal)
  Complex to Real-Imag/1 -> Fourier1/1(signal)

== system power_wind_dfig/Wind Turbine Protection/Protection System/AC Voltage Protection/Voltage Measurement/magnitude2 ==
  In1 : Inport
  Complex to Real-Imag : ComplexToRealImag
  Fourier1 : Subsystem  mask(Fourier analyser){f1=Freq, n=0}
      mask prompts: f1 "Fundamental frequency f1 (Hz):"; n "Harmonic n (0=DC; 1=fundamental; 2=2nd harm;  ...) :"
      mask help: The Fourier block performs a Fourier analysis of the input signal over a running window of one cycle of the fundamental frequency. First and second outputs return respectively the magnitude and phase (degrees) of the harmonic component specified.
      mask init:
      | k=2-(n==0);
      mask Help: helpview(psbhelp)
  Fourier2 : Subsystem  mask(Fourier analyser){f1=Freq, n=0}
      mask prompts: f1 "Fundamental frequency f1 (Hz):"; n "Harmonic n (0=DC; 1=fundamental; 2=2nd harm;  ...) :"
      mask help: The Fourier block performs a Fourier analysis of the input signal over a running window of one cycle of the fundamental frequency. First and second outputs return respectively the magnitude and phase (degrees) of the harmonic component specified.
      mask init:
      | k=2-(n==0);
      mask Help: helpview(psbhelp)
  Math Function : Math  Operator=hypot  SaturateOnIntegerOverflow=on
  Terminator : Terminator
  Terminator1 : Terminator
  Out1 : Outport
  wires:
  Complex to Real-Imag/1 -> Fourier1/1(signal)
  Complex to Real-Imag/2 -> Fourier2/1(signal)
  Fourier1/2(angle) -> Terminator/1
  Fourier2/2(angle) -> Terminator1/1
  Fourier1/1(magnitude) -> Math Function/1
  Fourier2/1(magnitude) -> Math Function/2
  Math Function/1 -> Out1/1
  In1/1 -> Complex to Real-Imag/1

== system power_wind_dfig/Plant 2 MVA/Plant & Motor Protection/AC Current Protection/Current Measurement/magnitude/Fourier1 ==
  signal : Inport
  Constant : Constant  Value=0
  Fcn : Fcn  Expr=u^2
  Fcn1 : Fcn  Expr=u^2
  Fcn2 : Fcn  Expr=sqrt(u)
  Fcn3 : Fcn  Expr=180/pi*atan2(u[2],u[1])
  Gain1 : Gain  Gain=k*f1  SaturateOnIntegerOverflow=on  OutDataTypeStr=Inherit: Same as input  ParamDataTypeStr=Inherit: Same as input
  Integ2 : Integrator  InitialConditionSource=external
  Mux : Mux  Inputs=2
  Product : Product  SaturateOnIntegerOverflow=on  InputSameDT=on  OutDataTypeStr=Inherit: Same as first input
  Product1 : Product  SaturateOnIntegerOverflow=on  InputSameDT=on  OutDataTypeStr=Inherit: Same as first input
  Sum : Sum  SaturateOnIntegerOverflow=on  InputSameDT=on  OutDataTypeStr=Inherit: Same as first input
  Sum1 : Sum  Inputs=+-  SaturateOnIntegerOverflow=on  InputSameDT=on  OutDataTypeStr=Inherit: Same as first input
  Sum2 : Sum  Inputs=+-  SaturateOnIntegerOverflow=on  InputSameDT=on  OutDataTypeStr=Inherit: Same as first input
  T : TransportDelay  DelayTime=1/f1  BufferSize=2048
  T1 : TransportDelay  DelayTime=1/f1  BufferSize=2048
  cos(nwt) : Sin  Frequency=2*pi*n*f1  Phase=pi/2  SampleTime=0
  integ1 : Integrator  InitialConditionSource=external
  sin(nwt) : Sin  Frequency=2*pi*n*f1  SampleTime=0
  magnitude : Outport  InitialOutput=0
  angle : Outport  Port=2  InitialOutput=0
  wires:
  Constant/1 -> integ1/2, Integ2/2
  Sum/1 -> Fcn2/1
  Fcn/1 -> Sum/1
  Fcn1/1 -> Sum/2
  Mux/1 -> Fcn3/1
  Fcn3/1 -> angle/1
  sin(nwt)/1 -> Product/1
  cos(nwt)/1 -> Product1/2
  Product/1 -> integ1/1
  Product1/1 -> Integ2/1
  T/1 -> Sum1/2
  T1/1 -> Sum2/2
  integ1/1 -> Sum1/1, T/1
  Integ2/1 -> T1/1, Sum2/1
  Sum2/1 -> Fcn1/1, Mux/2
  Sum1/1 -> Fcn/1, Mux/1
  signal/1 -> Gain1/1
  Gain1/1 -> Product/2, Product1/1
  Fcn2/1 -> magnitude/1

== system power_wind_dfig/Plant 2 MVA/Plant & Motor Protection/AC Current Protection/Current Measurement/magnitude/Fourier2 ==
  signal : Inport
  Constant : Constant  Value=0
  Fcn : Fcn  Expr=u^2
  Fcn1 : Fcn  Expr=u^2
  Fcn2 : Fcn  Expr=sqrt(u)
  Fcn3 : Fcn  Expr=180/pi*atan2(u[2],u[1])
  Gain1 : Gain  Gain=k*f1  SaturateOnIntegerOverflow=on  OutDataTypeStr=Inherit: Same as input  ParamDataTypeStr=Inherit: Same as input
  Integ2 : Integrator  InitialConditionSource=external
  Mux : Mux  Inputs=2
  Product : Product  SaturateOnIntegerOverflow=on  InputSameDT=on  OutDataTypeStr=Inherit: Same as first input
  Product1 : Product  SaturateOnIntegerOverflow=on  InputSameDT=on  OutDataTypeStr=Inherit: Same as first input
  Sum : Sum  SaturateOnIntegerOverflow=on  InputSameDT=on  OutDataTypeStr=Inherit: Same as first input
  Sum1 : Sum  Inputs=+-  SaturateOnIntegerOverflow=on  InputSameDT=on  OutDataTypeStr=Inherit: Same as first input
  Sum2 : Sum  Inputs=+-  SaturateOnIntegerOverflow=on  InputSameDT=on  OutDataTypeStr=Inherit: Same as first input
  T : TransportDelay  DelayTime=1/f1  BufferSize=2048
  T1 : TransportDelay  DelayTime=1/f1  BufferSize=2048
  cos(nwt) : Sin  Frequency=2*pi*n*f1  Phase=pi/2  SampleTime=0
  integ1 : Integrator  InitialConditionSource=external
  sin(nwt) : Sin  Frequency=2*pi*n*f1  SampleTime=0
  magnitude : Outport  InitialOutput=0
  angle : Outport  Port=2  InitialOutput=0
  wires:
  Fcn2/1 -> magnitude/1
  Gain1/1 -> Product1/1, Product/2
  signal/1 -> Gain1/1
  Sum1/1 -> Mux/1, Fcn/1
  Sum2/1 -> Mux/2, Fcn1/1
  Integ2/1 -> Sum2/1, T1/1
  integ1/1 -> T/1, Sum1/1
  T1/1 -> Sum2/2
  T/1 -> Sum1/2
  Product1/1 -> Integ2/1
  Product/1 -> integ1/1
  cos(nwt)/1 -> Product1/2
  sin(nwt)/1 -> Product/1
  Fcn3/1 -> angle/1
  Mux/1 -> Fcn3/1
  Fcn1/1 -> Sum/2
  Fcn/1 -> Sum/1
  Sum/1 -> Fcn2/1
  Constant/1 -> Integ2/2, integ1/2

== system power_wind_dfig/Plant 2 MVA/Plant & Motor Protection/AC Current Protection/Current Measurement/magnitude1/Fourier1 ==
  signal : Inport
  Constant : Constant  Value=0
  Fcn : Fcn  Expr=u^2
  Fcn1 : Fcn  Expr=u^2
  Fcn2 : Fcn  Expr=sqrt(u)
  Fcn3 : Fcn  Expr=180/pi*atan2(u[2],u[1])
  Gain1 : Gain  Gain=k*f1  SaturateOnIntegerOverflow=on  OutDataTypeStr=Inherit: Same as input  ParamDataTypeStr=Inherit: Same as input
  Integ2 : Integrator  InitialConditionSource=external
  Mux : Mux  Inputs=2
  Product : Product  SaturateOnIntegerOverflow=on  InputSameDT=on  OutDataTypeStr=Inherit: Same as first input
  Product1 : Product  SaturateOnIntegerOverflow=on  InputSameDT=on  OutDataTypeStr=Inherit: Same as first input
  Sum : Sum  SaturateOnIntegerOverflow=on  InputSameDT=on  OutDataTypeStr=Inherit: Same as first input
  Sum1 : Sum  Inputs=+-  SaturateOnIntegerOverflow=on  InputSameDT=on  OutDataTypeStr=Inherit: Same as first input
  Sum2 : Sum  Inputs=+-  SaturateOnIntegerOverflow=on  InputSameDT=on  OutDataTypeStr=Inherit: Same as first input
  T : TransportDelay  DelayTime=1/f1  BufferSize=2048
  T1 : TransportDelay  DelayTime=1/f1  BufferSize=2048
  cos(nwt) : Sin  Frequency=2*pi*n*f1  Phase=pi/2  SampleTime=0
  integ1 : Integrator  InitialConditionSource=external
  sin(nwt) : Sin  Frequency=2*pi*n*f1  SampleTime=0
  magnitude : Outport  InitialOutput=0
  angle : Outport  Port=2  InitialOutput=0
  wires:
  Fcn2/1 -> magnitude/1
  Gain1/1 -> Product1/1, Product/2
  signal/1 -> Gain1/1
  Sum1/1 -> Mux/1, Fcn/1
  Sum2/1 -> Mux/2, Fcn1/1
  Integ2/1 -> Sum2/1, T1/1
  integ1/1 -> T/1, Sum1/1
  T1/1 -> Sum2/2
  T/1 -> Sum1/2
  Product1/1 -> Integ2/1
  Product/1 -> integ1/1
  cos(nwt)/1 -> Product1/2
  sin(nwt)/1 -> Product/1
  Fcn3/1 -> angle/1
  Mux/1 -> Fcn3/1
  Fcn1/1 -> Sum/2
  Fcn/1 -> Sum/1
  Sum/1 -> Fcn2/1
  Constant/1 -> Integ2/2, integ1/2

== system power_wind_dfig/Plant 2 MVA/Plant & Motor Protection/AC Current Protection/Current Measurement/magnitude1/Fourier2 ==
  signal : Inport
  Constant : Constant  Value=0
  Fcn : Fcn  Expr=u^2
  Fcn1 : Fcn  Expr=u^2
  Fcn2 : Fcn  Expr=sqrt(u)
  Fcn3 : Fcn  Expr=180/pi*atan2(u[2],u[1])
  Gain1 : Gain  Gain=k*f1  SaturateOnIntegerOverflow=on  OutDataTypeStr=Inherit: Same as input  ParamDataTypeStr=Inherit: Same as input
  Integ2 : Integrator  InitialConditionSource=external
  Mux : Mux  Inputs=2
  Product : Product  SaturateOnIntegerOverflow=on  InputSameDT=on  OutDataTypeStr=Inherit: Same as first input
  Product1 : Product  SaturateOnIntegerOverflow=on  InputSameDT=on  OutDataTypeStr=Inherit: Same as first input
  Sum : Sum  SaturateOnIntegerOverflow=on  InputSameDT=on  OutDataTypeStr=Inherit: Same as first input
  Sum1 : Sum  Inputs=+-  SaturateOnIntegerOverflow=on  InputSameDT=on  OutDataTypeStr=Inherit: Same as first input
  Sum2 : Sum  Inputs=+-  SaturateOnIntegerOverflow=on  InputSameDT=on  OutDataTypeStr=Inherit: Same as first input
  T : TransportDelay  DelayTime=1/f1  BufferSize=2048
  T1 : TransportDelay  DelayTime=1/f1  BufferSize=2048
  cos(nwt) : Sin  Frequency=2*pi*n*f1  Phase=pi/2  SampleTime=0
  integ1 : Integrator  InitialConditionSource=external
  sin(nwt) : Sin  Frequency=2*pi*n*f1  SampleTime=0
  magnitude : Outport  InitialOutput=0
  angle : Outport  Port=2  InitialOutput=0
  wires:
  Constant/1 -> integ1/2, Integ2/2
  Sum/1 -> Fcn2/1
  Fcn/1 -> Sum/1
  Fcn1/1 -> Sum/2
  Mux/1 -> Fcn3/1
  Fcn3/1 -> angle/1
  sin(nwt)/1 -> Product/1
  cos(nwt)/1 -> Product1/2
  Product/1 -> integ1/1
  Product1/1 -> Integ2/1
  T/1 -> Sum1/2
  T1/1 -> Sum2/2
  integ1/1 -> Sum1/1, T/1
  Integ2/1 -> T1/1, Sum2/1
  Sum2/1 -> Fcn1/1, Mux/2
  Sum1/1 -> Fcn/1, Mux/1
  signal/1 -> Gain1/1
  Gain1/1 -> Product/2, Product1/1
  Fcn2/1 -> magnitude/1

== system power_wind_dfig/Plant 2 MVA/Plant & Motor Protection/AC Voltage Protection/Voltage Measurement/magnitude/Fourier1 ==
  signal : Inport
  Constant : Constant  Value=0
  Fcn : Fcn  Expr=u^2
  Fcn1 : Fcn  Expr=u^2
  Fcn2 : Fcn  Expr=sqrt(u)
  Fcn3 : Fcn  Expr=180/pi*atan2(u[2],u[1])
  Gain1 : Gain  Gain=k*f1  SaturateOnIntegerOverflow=on  OutDataTypeStr=Inherit: Same as input  ParamDataTypeStr=Inherit: Same as input
  Integ2 : Integrator  InitialConditionSource=external
  Mux : Mux  Inputs=2
  Product : Product  SaturateOnIntegerOverflow=on  InputSameDT=on  OutDataTypeStr=Inherit: Same as first input
  Product1 : Product  SaturateOnIntegerOverflow=on  InputSameDT=on  OutDataTypeStr=Inherit: Same as first input
  Sum : Sum  SaturateOnIntegerOverflow=on  InputSameDT=on  OutDataTypeStr=Inherit: Same as first input
  Sum1 : Sum  Inputs=+-  SaturateOnIntegerOverflow=on  InputSameDT=on  OutDataTypeStr=Inherit: Same as first input
  Sum2 : Sum  Inputs=+-  SaturateOnIntegerOverflow=on  InputSameDT=on  OutDataTypeStr=Inherit: Same as first input
  T : TransportDelay  DelayTime=1/f1  BufferSize=2048
  T1 : TransportDelay  DelayTime=1/f1  BufferSize=2048
  cos(nwt) : Sin  Frequency=2*pi*n*f1  Phase=pi/2  SampleTime=0
  integ1 : Integrator  InitialConditionSource=external
  sin(nwt) : Sin  Frequency=2*pi*n*f1  SampleTime=0
  magnitude : Outport  InitialOutput=0
  angle : Outport  Port=2  InitialOutput=0
  wires:
  Constant/1 -> integ1/2, Integ2/2
  Sum/1 -> Fcn2/1
  Fcn/1 -> Sum/1
  Fcn1/1 -> Sum/2
  Mux/1 -> Fcn3/1
  Fcn3/1 -> angle/1
  sin(nwt)/1 -> Product/1
  cos(nwt)/1 -> Product1/2
  Product/1 -> integ1/1
  Product1/1 -> Integ2/1
  T/1 -> Sum1/2
  T1/1 -> Sum2/2
  integ1/1 -> Sum1/1, T/1
  Integ2/1 -> T1/1, Sum2/1
  Sum2/1 -> Fcn1/1, Mux/2
  Sum1/1 -> Fcn/1, Mux/1
  signal/1 -> Gain1/1
  Gain1/1 -> Product/2, Product1/1
  Fcn2/1 -> magnitude/1

== system power_wind_dfig/Plant 2 MVA/Plant & Motor Protection/AC Voltage Protection/Voltage Measurement/magnitude/Fourier2 ==
  signal : Inport
  Constant : Constant  Value=0
  Fcn : Fcn  Expr=u^2
  Fcn1 : Fcn  Expr=u^2
  Fcn2 : Fcn  Expr=sqrt(u)
  Fcn3 : Fcn  Expr=180/pi*atan2(u[2],u[1])
  Gain1 : Gain  Gain=k*f1  SaturateOnIntegerOverflow=on  OutDataTypeStr=Inherit: Same as input  ParamDataTypeStr=Inherit: Same as input
  Integ2 : Integrator  InitialConditionSource=external
  Mux : Mux  Inputs=2
  Product : Product  SaturateOnIntegerOverflow=on  InputSameDT=on  OutDataTypeStr=Inherit: Same as first input
  Product1 : Product  SaturateOnIntegerOverflow=on  InputSameDT=on  OutDataTypeStr=Inherit: Same as first input
  Sum : Sum  SaturateOnIntegerOverflow=on  InputSameDT=on  OutDataTypeStr=Inherit: Same as first input
  Sum1 : Sum  Inputs=+-  SaturateOnIntegerOverflow=on  InputSameDT=on  OutDataTypeStr=Inherit: Same as first input
  Sum2 : Sum  Inputs=+-  SaturateOnIntegerOverflow=on  InputSameDT=on  OutDataTypeStr=Inherit: Same as first input
  T : TransportDelay  DelayTime=1/f1  BufferSize=2048
  T1 : TransportDelay  DelayTime=1/f1  BufferSize=2048
  cos(nwt) : Sin  Frequency=2*pi*n*f1  Phase=pi/2  SampleTime=0
  integ1 : Integrator  InitialConditionSource=external
  sin(nwt) : Sin  Frequency=2*pi*n*f1  SampleTime=0
  magnitude : Outport  InitialOutput=0
  angle : Outport  Port=2  InitialOutput=0
  wires:
  Fcn2/1 -> magnitude/1
  Gain1/1 -> Product1/1, Product/2
  signal/1 -> Gain1/1
  Sum1/1 -> Mux/1, Fcn/1
  Sum2/1 -> Mux/2, Fcn1/1
  Integ2/1 -> Sum2/1, T1/1
  integ1/1 -> T/1, Sum1/1
  T1/1 -> Sum2/2
  T/1 -> Sum1/2
  Product1/1 -> Integ2/1
  Product/1 -> integ1/1
  cos(nwt)/1 -> Product1/2
  sin(nwt)/1 -> Product/1
  Fcn3/1 -> angle/1
  Mux/1 -> Fcn3/1
  Fcn1/1 -> Sum/2
  Fcn/1 -> Sum/1
  Sum/1 -> Fcn2/1
  Constant/1 -> Integ2/2, integ1/2

== system power_wind_dfig/Plant 2 MVA/Plant & Motor Protection/AC Voltage Protection/Voltage Measurement/magnitude1/Fourier1 ==
  signal : Inport
  Constant : Constant  Value=0
  Fcn : Fcn  Expr=u^2
  Fcn1 : Fcn  Expr=u^2
  Fcn2 : Fcn  Expr=sqrt(u)
  Fcn3 : Fcn  Expr=180/pi*atan2(u[2],u[1])
  Gain1 : Gain  Gain=k*f1  SaturateOnIntegerOverflow=on  OutDataTypeStr=Inherit: Same as input  ParamDataTypeStr=Inherit: Same as input
  Integ2 : Integrator  InitialConditionSource=external
  Mux : Mux  Inputs=2
  Product : Product  SaturateOnIntegerOverflow=on  InputSameDT=on  OutDataTypeStr=Inherit: Same as first input
  Product1 : Product  SaturateOnIntegerOverflow=on  InputSameDT=on  OutDataTypeStr=Inherit: Same as first input
  Sum : Sum  SaturateOnIntegerOverflow=on  InputSameDT=on  OutDataTypeStr=Inherit: Same as first input
  Sum1 : Sum  Inputs=+-  SaturateOnIntegerOverflow=on  InputSameDT=on  OutDataTypeStr=Inherit: Same as first input
  Sum2 : Sum  Inputs=+-  SaturateOnIntegerOverflow=on  InputSameDT=on  OutDataTypeStr=Inherit: Same as first input
  T : TransportDelay  DelayTime=1/f1  BufferSize=2048
  T1 : TransportDelay  DelayTime=1/f1  BufferSize=2048
  cos(nwt) : Sin  Frequency=2*pi*n*f1  Phase=pi/2  SampleTime=0
  integ1 : Integrator  InitialConditionSource=external
  sin(nwt) : Sin  Frequency=2*pi*n*f1  SampleTime=0
  magnitude : Outport  InitialOutput=0
  angle : Outport  Port=2  InitialOutput=0
  wires:
  Fcn2/1 -> magnitude/1
  Gain1/1 -> Product1/1, Product/2
  signal/1 -> Gain1/1
  Sum1/1 -> Mux/1, Fcn/1
  Sum2/1 -> Mux/2, Fcn1/1
  Integ2/1 -> Sum2/1, T1/1
  integ1/1 -> T/1, Sum1/1
  T1/1 -> Sum2/2
  T/1 -> Sum1/2
  Product1/1 -> Integ2/1
  Product/1 -> integ1/1
  cos(nwt)/1 -> Product1/2
  sin(nwt)/1 -> Product/1
  Fcn3/1 -> angle/1
  Mux/1 -> Fcn3/1
  Fcn1/1 -> Sum/2
  Fcn/1 -> Sum/1
  Sum/1 -> Fcn2/1
  Constant/1 -> Integ2/2, integ1/2

== system power_wind_dfig/Plant 2 MVA/Plant & Motor Protection/AC Voltage Protection/Voltage Measurement/magnitude1/Fourier2 ==
  signal : Inport
  Constant : Constant  Value=0
  Fcn : Fcn  Expr=u^2
  Fcn1 : Fcn  Expr=u^2
  Fcn2 : Fcn  Expr=sqrt(u)
  Fcn3 : Fcn  Expr=180/pi*atan2(u[2],u[1])
  Gain1 : Gain  Gain=k*f1  SaturateOnIntegerOverflow=on  OutDataTypeStr=Inherit: Same as input  ParamDataTypeStr=Inherit: Same as input
  Integ2 : Integrator  InitialConditionSource=external
  Mux : Mux  Inputs=2
  Product : Product  SaturateOnIntegerOverflow=on  InputSameDT=on  OutDataTypeStr=Inherit: Same as first input
  Product1 : Product  SaturateOnIntegerOverflow=on  InputSameDT=on  OutDataTypeStr=Inherit: Same as first input
  Sum : Sum  SaturateOnIntegerOverflow=on  InputSameDT=on  OutDataTypeStr=Inherit: Same as first input
  Sum1 : Sum  Inputs=+-  SaturateOnIntegerOverflow=on  InputSameDT=on  OutDataTypeStr=Inherit: Same as first input
  Sum2 : Sum  Inputs=+-  SaturateOnIntegerOverflow=on  InputSameDT=on  OutDataTypeStr=Inherit: Same as first input
  T : TransportDelay  DelayTime=1/f1  BufferSize=2048
  T1 : TransportDelay  DelayTime=1/f1  BufferSize=2048
  cos(nwt) : Sin  Frequency=2*pi*n*f1  Phase=pi/2  SampleTime=0
  integ1 : Integrator  InitialConditionSource=external
  sin(nwt) : Sin  Frequency=2*pi*n*f1  SampleTime=0
  magnitude : Outport  InitialOutput=0
  angle : Outport  Port=2  InitialOutput=0
  wires:
  Constant/1 -> integ1/2, Integ2/2
  Sum/1 -> Fcn2/1
  Fcn/1 -> Sum/1
  Fcn1/1 -> Sum/2
  Mux/1 -> Fcn3/1
  Fcn3/1 -> angle/1
  sin(nwt)/1 -> Product/1
  cos(nwt)/1 -> Product1/2
  Product/1 -> integ1/1
  Product1/1 -> Integ2/1
  T/1 -> Sum1/2
  T1/1 -> Sum2/2
  integ1/1 -> Sum1/1, T/1
  Integ2/1 -> T1/1, Sum2/1
  Sum2/1 -> Fcn1/1, Mux/2
  Sum1/1 -> Fcn/1, Mux/1
  signal/1 -> Gain1/1
  Gain1/1 -> Product/2, Product1/1
  Fcn2/1 -> magnitude/1
